simulink model "BLDC_Motor"  (R2020b)
settings: Solver=VariableStepAuto  StartTime=0.0  StopTime=10.0  RelTol=1e-3
values from neighbouring files (symbols this model uses):
  Kd = 0.1782    [initial_values.m]
  Ki = 413.7806    [initial_values.m]
  Kp = 6.0449    [initial_values.m]
settings Model: Creator=shubham sharma  LastModifiedBy=shubham sharma

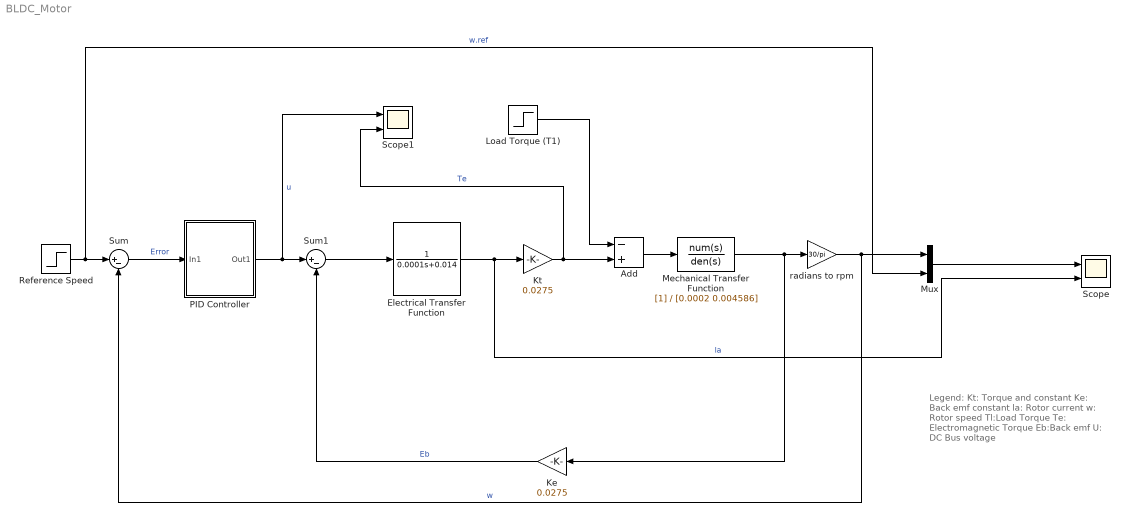
== system BLDC_Motor ==
  note: Legend:
      | Kt: Torque and constant
      | Ke: Back emf constant
      | la: Rotor current
      | w: Rotor speed
      | Tl:Load Torque
      | Te: Electromagnetic Torque
      | Eb:Back emf
      | U: DC Bus voltage
  Add : Sum  Inputs=-+
  Electrical Transfer Function : TransferFcn  Denominator=[0.0001 0.014]
  Ke : Gain  Gain=0.0275
  Kt : Gain  Gain=0.0275
  Load Torque (T1) : Step  Time=0.1  After=10  SampleTime=0
  Mechanical Transfer Function : TransferFcn  Denominator=[0.0002 0.004586]
  Mux : Mux  Inputs=2
  PID Controller : Subsystem
  Reference Speed : Step  Time=0  After=1500  SampleTime=0
  Scope : Scope  NumInputPorts=2
  Scope1 : Scope  NumInputPorts=2
  Sum : Sum  Inputs=|+-
  Sum1 : Sum  Inputs=|+-
  radians to rpm : Gain  Gain=30/pi
  wires:
  Reference Speed/1 -> Sum/1, Mux/2  "w.ref"
  Sum/1 -> PID Controller/1(In1)  "Error"
  PID Controller/1(Out1) -> Scope1/1, Sum1/1  "u"
  Ke/1 -> Sum1/2  "Eb"
  Sum1/1 -> Electrical Transfer Function/1
  Electrical Transfer Function/1 -> Scope/2, Kt/1  "la"
  Kt/1 -> Scope1/2, Add/2  "Te"
  Load Torque (T1)/1 -> Add/1
  Add/1 -> Mechanical Transfer Function/1
  Mechanical Transfer Function/1 -> Ke/1, radians to rpm/1
  Mux/1 -> Scope/1
  radians to rpm/1 -> Sum/2, Mux/1  "w"

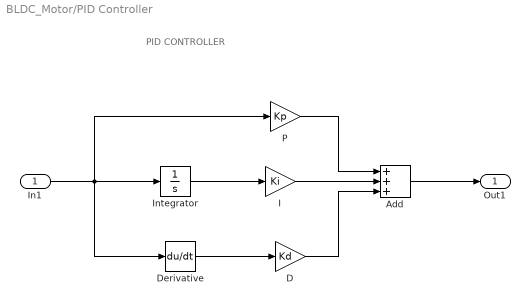
== system BLDC_Motor/PID Controller ==
  note: PID CONTROLLER
  In1 : Inport
  Add : Sum  Inputs=+++
  D : Gain  Gain=Kd
  Derivative : Derivative
  I : Gain  Gain=Ki
  Integrator : Integrator
  P : Gain  Gain=Kp
  Out1 : Outport
  wires:
  In1/1 -> Integrator/1, Derivative/1, P/1
  Integrator/1 -> I/1
  I/1 -> Add/2
  Derivative/1 -> D/1
  D/1 -> Add/3
  P/1 -> Add/1
  Add/1 -> Out1/1
